simulink model "positioncontrolbasisagent"  (Simulink 6.2)
settings: Solver=ode45  StartTime=0.0  StopTime=10.0  RelTol=1e-3
settings Model: LastModifiedBy=suarezjl
settings DebuggingCC: SolverPrmCheckMsg=warning

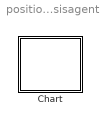
== system positioncontrolbasisagent ==
  Chart : Stateflow chart

== stateflow chart Chart ==
  state Initialize
    Aquateen\ControlBasisModule\PositionControlBasis\PositionCB.Initialize()
    Aquateen\ControlBasisModule\HP3JCAgent\HP3JC.connect_Initialize()
    Aquateen\ControlBasisModule\HP3JCAgent\HP3JC.servo_ServoOn()
    Aquateen\ControlBasisModule\HP3JCAgent\HP3JC.job_SelectJob()
    Aquateen\ControlBasisModule\HP3JCAgent\HP3JC.job_StartJob()
  state ComputeBasis
    Aquateen\ControlBasisModule\HP3JCAgent\HP3JC.read_CurrentPosition()
    Aquateen\ControlBasisModule\PositionControlBasis\PositionCB.ComputeControlBasis()
    Aquateen\ControlBasisModule\HP3JCAgent\HP3JC.move_JointAngles()
  state EmptyContent
    Aquateen\ControlBasisModule\HP3JCAgent\HP3JC.error_ClearError()
    Aquateen\ControlBasisModule\HP3JCAgent\HP3JC.error_ClearAlarm()
    Aquateen\ControlBasisModule\HP3JCAgent\HP3JC.job_SelectJob()
    Aquateen\ControlBasisModule\HP3JCAgent\HP3JC.job_StartJob()
    Aquateen\ControlBasisModule\PositionControlBasis\StateMachine.Wait(2000)
    Aquateen\ControlBasisModule\HP3JCAgent\HP3JC.connect_Disconnect()
  (default) -> Initialize : Start
  ComputeBasis -> ComputeBasis [order 1] : Default
  Initialize -> ComputeBasis : Always
  ComputeBasis -> EmptyContent [order 2] : Signal="End"
